simulink model "Problem_7"  (R2020a)
settings: Solver=VariableStepAuto  StartTime=0.0  StopTime=10.0  RelTol=1e-3
settings Model: Creator=user  LastModifiedBy=user

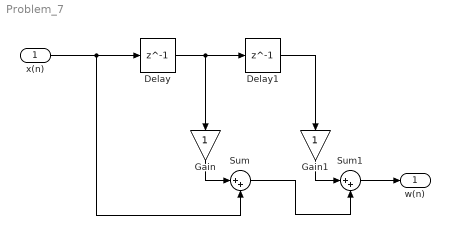
== system Problem_7 ==
  x(n) : Inport
  Delay : Delay  DelayLength=1
  Delay1 : Delay  DelayLength=1
  Gain : Gain
  Gain1 : Gain
  Sum : Sum  Inputs=|++
  Sum1 : Sum  Inputs=|++
  w(n) : Outport
  wires:
  Delay/1 -> Delay1/1, Gain/1
  x(n)/1 -> Sum/2, Delay/1
  Delay1/1 -> Gain1/1
  Gain/1 -> Sum/1
  Sum/1 -> Sum1/2
  Gain1/1 -> Sum1/1
  Sum1/1 -> w(n)/1
